simulink model "Record"  (Simulink 7.5)
settings: Solver=ode45  StartTime=0.0  StopTime=20  RelTol=1e-3
settings Model: Creator=ftheis  LastModifiedBy=ftheis
settings DataIOCC: TimeSaveName=time

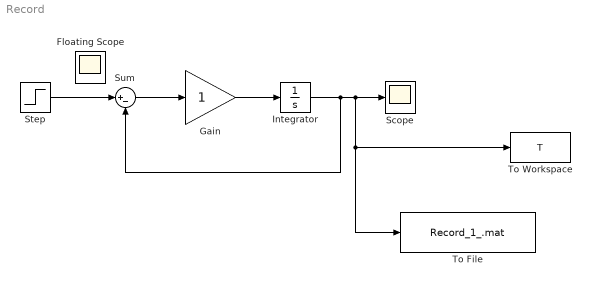
== system Record ==
  Gain : Gain  ParameterDataType=fixdt(1, 16)  ParameterScaling=2^0  OutDataType=fixdt(1, 16)  OutScaling=2^0
  Integrator : Integrator  InitialCondition=20
  Scope : Scope
      settings: YMin=28.5  YMax=31.5
  Step : Step  Time=3  Before=20  After=30  SampleTime=0
  Sum : Sum  Inputs=|+-  OutDataType=fixdt(1, 16)  OutScaling=2^0
  To File : ToFile  Filename=Record_1_.mat  MatrixName=Tfile  SaveFormat=Timeseries
  To Workspace : ToWorkspace  VariableName=T  SampleTime=-1  SaveFormat=Array
  Floating Scope : Scope
      settings: Floating=on  YMin=10  YMax=40
  wires:
  Step/1 -> Sum/1
  Sum/1 -> Gain/1
  Gain/1 -> Integrator/1
  Integrator/1 -> Sum/2, Scope/1, To File/1, To Workspace/1
